simulink model "OT_01_Motor_continuo"  (Simulink 7.7)
settings: Solver=ode45  StartTime=0.0  StopTime=20.0  RelTol=1e-3
values from neighbouring files (symbols this model uses):
  alfa = 1    [OT_01_inicial.m]
  beta = 1    [OT_01_inicial.m]
undefined symbols (not defined in the file or in its folder): a, b, k, magnitude
settings Model: Creator=vanderleiparro  LastModifiedBy=vanderleiparro
settings DataIOCC: SignalLoggingName=sigsOut
settings DebuggingCC: SaveWithParameterizedLinksMsg=none  SignalResolutionControl=TryResolveAllWithWarning  SolverPrmCheckMsg=none  MultiTaskDSMMsg=warning  MultiTaskCondExecSysMsg=none  StrictBusMsg=None
settings HardwareCC: TargetUnknown=on
settings RTWCC: IncludeERTFirstTime=on

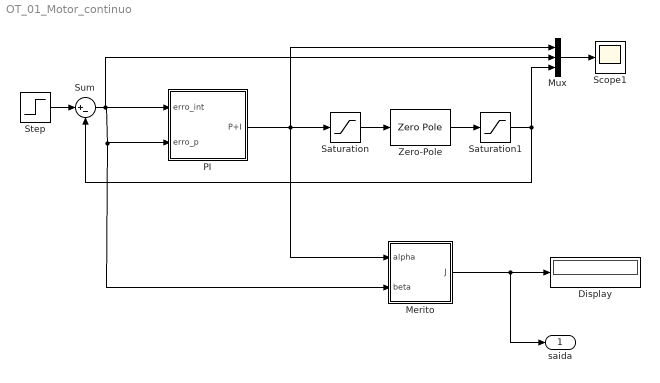
== system OT_01_Motor_continuo ==
  Display : Display
  Merito : Subsystem
  Mux : Mux  Inputs=3
  PI : Subsystem
  Saturation : Saturate  UpperLimit=10  LowerLimit=-10
  Saturation1 : Saturate  UpperLimit=10  LowerLimit=-10
  Scope1 : Scope
      settings: YMin=-1  YMax=1.75
  Step : Step  SampleTime=0
  Sum : Sum  Inputs=|+-  SaturateOnIntegerOverflow=on
  Zero-Pole : ZeroPole  Zeros=[]  Poles=[0 -2]
  saida : Outport
  wires:
  Sum/1 -> PI/1(erro_int), Mux/2, Merito/2(beta), PI/2(erro_p)
  Step/1 -> Sum/1
  Saturation/1 -> Zero-Pole/1
  Merito/1(J) -> Display/1, saida/1
  Zero-Pole/1 -> Saturation1/1
  Saturation1/1 -> Sum/2, Mux/3
  PI/1(P+I) -> Saturation/1, Merito/1(alpha), Mux/1
  Mux/1 -> Scope1/1

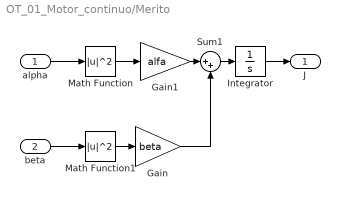
== system OT_01_Motor_continuo/Merito ==
  alpha : Inport
  beta : Inport  Port=2
  Gain : Gain  Gain=beta  SaturateOnIntegerOverflow=on  OutDataTypeStr=Inherit: Same as input  ParamDataTypeStr=Inherit: Same as input
  Gain1 : Gain  Gain=alfa  SaturateOnIntegerOverflow=on  OutDataTypeStr=Inherit: Same as input  ParamDataTypeStr=Inherit: Same as input
  Integrator : Integrator
  Math Function : Math  Operator=magnitude^2  SaturateOnIntegerOverflow=on
  Math Function1 : Math  Operator=magnitude^2  SaturateOnIntegerOverflow=on
  Sum1 : Sum  Inputs=|++  SaturateOnIntegerOverflow=on
  J : Outport
  wires:
  Sum1/1 -> Integrator/1
  Math Function1/1 -> Gain/1
  Gain/1 -> Sum1/2
  Math Function/1 -> Gain1/1
  Gain1/1 -> Sum1/1
  alpha/1 -> Math Function/1
  beta/1 -> Math Function1/1
  Integrator/1 -> J/1

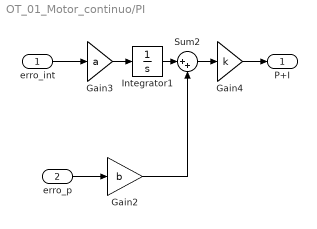
== system OT_01_Motor_continuo/PI ==
  erro_int : Inport
  erro_p : Inport  Port=2
  Gain2 : Gain  Gain=b  SaturateOnIntegerOverflow=on  OutDataTypeStr=Inherit: Same as input  ParamDataTypeStr=Inherit: Same as input
  Gain3 : Gain  Gain=a  SaturateOnIntegerOverflow=on  OutDataTypeStr=Inherit: Same as input  ParamDataTypeStr=Inherit: Same as input
  Gain4 : Gain  Gain=k  SaturateOnIntegerOverflow=on  OutDataTypeStr=Inherit: Same as input  ParamDataTypeStr=Inherit: Same as input
  Integrator1 : Integrator
  Sum2 : Sum  Inputs=|++  SaturateOnIntegerOverflow=on
  P+I : Outport
  wires:
  Gain2/1 -> Sum2/2
  Integrator1/1 -> Sum2/1
  Gain3/1 -> Integrator1/1
  Sum2/1 -> Gain4/1
  erro_int/1 -> Gain3/1
  erro_p/1 -> Gain2/1
  Gain4/1 -> P+I/1
